simulink model "atrias_original"  (R2017a)
settings: Solver=ode45  StartTime=0.0  StopTime=sim_t  RelTol=1e-6  EnableMultiTasking=on
values from neighbouring files (symbols this model uses):
  N = grid_slice*1000    [createGrid.m]
  nm = fn_set_vnmc_params(sm, sample_time)    [kernel_scores_NM_mismatch.m]    (also in main_ATRIAS_cluster.m)
  nmc_BLCtrlPar = nmc.BLCtrlPar    [kernel_scores_NM_mismatch.m]    (also in main_ATRIAS_cluster.m)
  nmc_FPCtrlPar = nmc.FPCtrlPar    [kernel_scores_NM_mismatch.m]    (also in main_ATRIAS_cluster.m)
  nmc_LLCtrlPar = nmc.LLCtrlPar    [kernel_scores_NM_mismatch.m]    (also in main_ATRIAS_cluster.m)
  nmc_StCtrlPar = nmc.StCtrlPar    [kernel_scores_NM_mismatch.m]    (also in main_ATRIAS_cluster.m)
  nmc_SwCtrlPar = nmc.SwCtrlPar    [kernel_scores_NM_mismatch.m]    (also in main_ATRIAS_cluster.m)
  nmc_TrCtrlPar = nmc.TrCtrlPar    [kernel_scores_NM_mismatch.m]    (also in main_ATRIAS_cluster.m)
  nStep_switchCtrl = 10    [main_ATRIAS_cluster.m]
  nStep_thr = 1000    [createSimInitial.m]    (also in main_ATRIAS_cluster.m)
  rc_CtrlPar = [rc.k_placement, rc.T_step, rc.Cd, rc.kpt, rc.kdt, rc.desired_theta, rc.desired_z, rc.kpz, rc.kdz]    [kernel_scores_NM_mismatch.m]    (also in main_ATRIAS_cluster.m)
  sm = fn_set_MechParams(sm)    [kernel_scores_NM_mismatch.m]    (also in main_ATRIAS_cluster.m = fn_set_MechParams(sm,perturb))
  test_VNMC = 1    [createSimInitial.m]    (also in main_ATRIAS_cluster.m = 0)
undefined symbols (not defined in the file or in its folder): delta_phi_max, delta_phi_max_buffer, delta_phi_min, DiscIntNeverNeededParam, Discrete, idc, initial_dx_estimate, initial_dy_estimate, initial_dz_estimate, initial_z_estimate, kd_shin_max, kd_shin_min, kd_splay_max, kd_splay_min, kd_thigh_max, kd_thigh_min, kp_shin_max, kp_shin_min, kp_splay_max, kp_splay_min, kp_thigh_max, kp_thigh_min, mc, min_splay_angle, min_splay_buffer, phi_shin_max, phi_shin_max_buffer, phi_shin_min, phi_shin_min_buffer, phi_thigh_max, phi_thigh_max_buffer, phi_thigh_min, phi_thigh_min_buffer, rad, rc, s, sample_time, sgn, sim_d, t_friction, Time, X, Y, Z
libraries: sm_lib x202, nesl_utility x122, simulink x77, simulink_extras x24, fl_lib x16, mblibv1 x4, ctrlSharedLib x4, commnoisgen2 x1, dspswit3 x1
(part 6 of 17)

== system atrias_original/control/RC control/State Estimation ==
  Right or Left [1/0] : Inport
  Torso Roll [rad rad/s] : Inport  Port=2
  Torso Pitch [rad rad/s] : Inport  Port=3
  Torso Yaw [rad rad/s] : Inport  Port=4
  Left Leg Sagittal Angle [rad rad/s] : Inport  Port=5
  Left Leg Roll [rad rad/s] : Inport  Port=6
  Left Leg Length [m m/s] : Inport  Port=7
  Right Leg Sagittal Angle [rad rad/s] : Inport  Port=8
  Right Leg Roll [rad rad/s] : Inport  Port=9
  Right Leg Length [m m/s] : Inport  Port=10
  Enable Kalman Filtering [1/0] : Inport  Port=11
  Right GRF [X Z] [N N] : Inport  Port=12
  Left GRF [X Z] [N N] : Inport  Port=13
  " Acceleration Measurement [m/s^2] x3" : Inport  Port=14
  Entering Stance [1/0] : Inport  Port=15
  Demux : Demux  Outputs=2
  Demux{1..7} (7 alike) : Demux  Outputs=3
  Demux11 : Demux  Outputs=2
  Demux8 : Demux  Outputs=2
  Discrete-Time Integrator : DiscreteIntegrator  InitialConditionSetting=State (most efficient)  SampleTime=-1  ICPrevOutput=DiscIntNeverNeededParam  ICPrevScaledInput=DiscIntNeverNeededParam
  From3 : From  Commented=on  GotoTag=RightLeftPrimary
  Gain : Gain  Gain=[1 1 0 1 1 0 1 1 0]
  Kalman Filtering : Subsystem
  Logical Operator1 : Logic  Operator=NOT  AllPortsSameDT=off  OutDataTypeStr=boolean
  Mux{,1,3,5,8..9,11..12} (8 alike) : Mux  Inputs=3
  Mux{2,4,6,10,13..20} (12 alike) : Mux  Inputs=2
  PositionUsingRobotGeometry : MATLAB Function  TreatAsAtomicUnit=on
  Product3 : Product
  Product4 : Product
  Selector : Selector  InputPortWidth=2  IndexOptions=Index vector (dialog)  Indices=[2]  OutputSizes=1
  Selector1 : Selector  InputPortWidth=2  IndexOptions=Index vector (dialog)  Indices=[2]  OutputSizes=1
  Selector2 : Selector  InputPortWidth=2  IndexOptions=Index vector (dialog)  Indices=[2]  OutputSizes=1
  Sum : Sum  Inputs=|++
  Switch : Switch  Criteria=u2 ~= 0
  Switch1 : Switch  Criteria=u2 ~= 0
  Switch2 : Switch  Criteria=u2 ~= 0
  Switch3 : Switch  Commented=on  Criteria=u2 ~= 0
  Terminator6 : Terminator
  X Kalman Output : Scope  NumInputPorts=3
  Y Kalman Output : Scope  NumInputPorts=3
  Z Kalman Output : Scope  NumInputPorts=3
  "[ddx, ddy, ddz]" : Selector  InputPortWidth=9  IndexOptions=Index vector (dialog)  Indices=[3 6 9]  OutputSizes=1
  "[x dx]" : Selector  InputPortWidth=9  IndexOptions=Index vector (dialog)  Indices=[1 2]  OutputSizes=1
  "[y dy]" : Selector  InputPortWidth=9  IndexOptions=Index vector (dialog)  Indices=[4 5]  OutputSizes=1
  "[z dz]" : Selector  InputPortWidth=9  IndexOptions=Index vector (dialog)  Indices=[7 8]  OutputSizes=1
  body frame : Selector  InputPortWidth=9  IndexOptions=Index vector (dialog)  Indices=[1 2 3]  OutputSizes=1
  body frame1 : Selector  InputPortWidth=9  IndexOptions=Index vector (dialog)  Indices=[1 2 3]  OutputSizes=1
  body frame{2..9} (8 alike) : Selector  InputPortWidth=9  IndexOptions=Index vector (dialog)  Indices=[4 5 6]  OutputSizes=1
  "Horizontal COM [m, m/s]" : Outport
  "Lateral COM [m, m/s]" : Outport  Port=2
  "Vertical COM [m, m/s]" : Outport  Port=3
  Pelvis to COM Position [m m m] : Outport  Port=4
  Pelvis to COM Velocity [m/s m/s m/s] : Outport  Port=5
  Primary Foot to COM Position [m m m] : Outport  Port=6
  Primary Foot to COM Velocity [m/s m/s m/s] : Outport  Port=7
  COM Acceleration [m/s^2] x3 : Outport  Port=8
  Secondary to COM Position [m m m] : Outport  Port=9  PortDimensions=3
  Secondary to COM Velocity [m/s m/s m/s] : Outport  Port=10  PortDimensions=3
  wires:
  Discrete-Time Integrator/1 -> Mux11/3
  Demux5/3 -> Mux12/1, Discrete-Time Integrator/1
  Demux5/2 -> Mux11/1
  Demux5/1 -> Mux13/1
  Demux4/3 -> Mux12/2
  Mux11/1 -> X Kalman Output/2
  Demux4/1 -> Mux13/2
  Demux4/2 -> Mux11/2
  Mux13/1 -> X Kalman Output/1
  Mux12/1 -> X Kalman Output/3
  Mux9/1 -> Mux3/2, Demux7/1, Kalman Filtering/10("Initial [y, dy, ddy] [m, m/s, m/s^2]")
  Mux8/1 -> Mux3/1, Demux5/1, Kalman Filtering/9("Initial [x, dx, ddx] [m, m/s, m/s^2]")
  "[ddx, ddy, ddz]"/1 -> COM Acceleration [m/s^2] x3/1
  Mux3/1 -> Gain/1
  Demux2/2 -> Mux9/3
  Demux2/1 -> Mux8/3
  Demux2/3 -> Mux/3
  " Acceleration Measurement [m/s^2] x3"/1 -> Demux2/1, Kalman Filtering/12(COM XYZ Acceleration [m/s^2] x3)
  Left Leg Sagittal Angle [rad rad/s]/1 -> PositionUsingRobotGeometry/5(left_leg_sagittal_angle)
  Left Leg Roll [rad rad/s]/1 -> PositionUsingRobotGeometry/6(left_leg_lateral_angle)
  Left Leg Length [m m/s]/1 -> PositionUsingRobotGeometry/7(left_leg_length)
  Right Leg Sagittal Angle [rad rad/s]/1 -> PositionUsingRobotGeometry/8(right_leg_sagittal_angle)
  Right Leg Roll [rad rad/s]/1 -> PositionUsingRobotGeometry/9(right_leg_lateral_angle)
  Right Leg Length [m m/s]/1 -> PositionUsingRobotGeometry/10(right_leg_length)
  Right or Left [1/0]/1 -> [RightLeftPrimary], PositionUsingRobotGeometry/1(right_left)
  Torso Roll [rad rad/s]/1 -> PositionUsingRobotGeometry/2(roll)
  Torso Yaw [rad rad/s]/1 -> PositionUsingRobotGeometry/4(yaw)
  Torso Pitch [rad rad/s]/1 -> PositionUsingRobotGeometry/3(pitch)
  Mux5/1 -> Switch/1
  Selector/1 -> Kalman Filtering/7(Right Vertical GRF [N])
  Selector1/1 -> Kalman Filtering/8(Left Vertical GRF [N])
  Product4/1 -> Sum/2, Selector1/1
  Product3/1 -> Sum/1, Selector/1
  Sum/1 -> Demux/1
  Enable Kalman Filtering [1/0]/1 -> Kalman Filtering/Enable, [EnableKalmanFiltering]
  Demux/1 -> Kalman Filtering/5(GRFx [N])
  Mux1/1 -> Terminator6/1
  PositionUsingRobotGeometry/12(dcom_pelvis) -> body frame1/1
  PositionUsingRobotGeometry/11(com_pelvis) -> body frame/1
  body frame/1 -> Pelvis to COM Position [m m m]/1
  body frame1/1 -> Pelvis to COM Velocity [m/s m/s m/s]/1
  PositionUsingRobotGeometry/7(lateral_com_position) -> Mux9/1
  "[z dz]"/1 -> "Vertical COM [m, m/s]"/1
  Switch/1 -> "[x dx]"/1, "[y dy]"/1, "[z dz]"/1, "[ddx, ddy, ddz]"/1
  "[y dy]"/1 -> "Lateral COM [m, m/s]"/1
  Demux/2 -> Kalman Filtering/6(GRFz [N])
  Kalman Filtering/1("[x, dx, ddx] [m/s, m/s^2]") -> Mux5/1, Demux4/1
  Kalman Filtering/3("[z, dz, ddz] [m, m/s, m/s^2]") -> Demux1/1, Mux5/3
  Kalman Filtering/2("[y, dy, ddy] [m/s, m/s^2]") -> Demux6/1, Mux5/2
  Kalman Filtering/5("[y, dy, ddy] uncertainty") -> Mux1/2
  Kalman Filtering/4("[x, dx, ddx] uncertainty") -> Mux1/1
  Kalman Filtering/6("[z, dz, ddz] uncertainty") -> Mux1/3
  PositionUsingRobotGeometry/9(vertical_com_position) -> Mux/1
  PositionUsingRobotGeometry/10(vertical_com_velocity) -> Mux/2
  Mux/1 -> Mux3/3, Demux3/1, Kalman Filtering/11("Initial [z, dz, ddz] [m m/s m/s^2]")
  PositionUsingRobotGeometry/8(lateral_com_velocity) -> Mux9/2
  PositionUsingRobotGeometry/6(horizontal_com_velocity) -> Mux8/2
  [RightLeftPrimary] -> Switch2/2
  Mux17/1 -> Switch2/3
  Mux16/1 -> Switch2/1
  Switch2/1 -> Demux11/1
  Demux11/2 -> Primary Foot to COM Velocity [m/s m/s m/s]/1
  Demux11/1 -> Primary Foot to COM Position [m m m]/1
  body frame2/1 -> Mux17/1
  body frame3/1 -> Mux17/2
  body frame5/1 -> Mux16/2
  body frame4/1 -> Mux16/1
  Entering Stance [1/0]/1 -> Kalman Filtering/13(Entering Stance [1/0])
  Mux4/1 -> Z Kalman Output/3
  Mux6/1 -> Z Kalman Output/1
  Demux1/2 -> Mux10/2
  Demux1/1 -> Mux6/2
  Mux10/1 -> Z Kalman Output/2
  Demux1/3 -> Mux4/2
  Demux3/1 -> Mux6/1
  Demux3/2 -> Mux10/1
  Demux3/3 -> Mux4/1
  Mux15/1 -> Y Kalman Output/3
  Mux18/1 -> Y Kalman Output/1
  Demux6/2 -> Mux14/2
  Demux6/1 -> Mux18/2
  Mux14/1 -> Y Kalman Output/2
  Demux6/3 -> Mux15/2
  Demux7/1 -> Mux18/1
  Demux7/2 -> Mux14/1
  Demux7/3 -> Mux15/1
  [EnableKalmanFiltering] -> Switch/2
  PositionUsingRobotGeometry/1(com_left_foot) -> body frame8/1, body frame2/1, Kalman Filtering/1("COM from Left Foot [body, yawed, global]")
  PositionUsingRobotGeometry/2(dcom_left_foot) -> body frame9/1, body frame3/1, Kalman Filtering/2("dCOM from Left Foot [body, yawed, global]")
  PositionUsingRobotGeometry/3(com_right_foot) -> body frame6/1, body frame4/1, Kalman Filtering/3("COM from Right Foot [body, yawed, global]")
  PositionUsingRobotGeometry/4(dcom_right_foot) -> Kalman Filtering/4("dCOM from Right Foot [body, yawed, global]"), body frame7/1, body frame5/1
  [RightLeftPrimary] -> Switch1/2
  Mux20/1 -> Switch1/3
  Mux19/1 -> Switch1/1
  Switch1/1 -> Demux8/1
  Demux8/2 -> Secondary to COM Velocity [m/s m/s m/s]/1
  Demux8/1 -> Secondary to COM Position [m m m]/1
  body frame6/1 -> Mux20/1
  body frame7/1 -> Mux20/2
  body frame9/1 -> Mux19/2
  body frame8/1 -> Mux19/1
  Gain/1 -> Switch/3
  From3/1 -> Switch3/2
  Logical Operator1/1 -> Product4/1
  Left GRF [X Z] [N N]/1 -> Product4/2
  Right GRF [X Z] [N N]/1 -> Product3/2
  [RightLeftPrimary] -> Logical Operator1/1, Product3/1
  Mux2/1 -> "Horizontal COM [m, m/s]"/1
  Selector2/1 -> Mux2/2
  "[x dx]"/1 -> Selector2/1
  PositionUsingRobotGeometry/5(horizontal_com_position) -> Mux2/1, Mux8/1

== system atrias_original/control/RC control/Step Count ==
  In1 : Inport
  Data Type Conversion : DataTypeConversion  OutDataTypeStr=uint32
  Sum1 : Sum  Inputs=|++
  Unit Delay : UnitDelay  SampleTime=-1
  step count : Scope
  Out1 : Outport
  wires:
  In1/1 -> Data Type Conversion/1
  Unit Delay/1 -> Sum1/2
  Sum1/1 -> Out1/1, Unit Delay/1, step count/1
  Data Type Conversion/1 -> Sum1/1

== system atrias_original/control/RC control/Swing ==
  desired_x : Inport
  EnteringStance : Inport  Port=2
  nstep : Inport  Port=3
  secondary_x : Inport  Port=4
  tSim : Inport  Port=5
  T_step : Inport  Port=6
  Enabled Subsystem : Subsystem  TreatAsAtomicUnit=on
  Hold Value1 : Subsystem  TreatAsAtomicUnit=on
  Sum5 : Sum  Inputs=|-+
  To Workspace1 : ToWorkspace  VariableName=nStep  SampleTime=-1
      settings: MaxDataPoints=1  Save2DSignal=2-D array (concatenate along first dimension)
  Unit Delay1 : UnitDelay  InitialCondition=0.4  SampleTime=sample_time
  swing_trajectory_regenerator : MATLAB Function  TreatAsAtomicUnit=on
  x : Outport
  xd : Outport  Port=2
  xdd : Outport  Port=3
  z : Outport  Port=4
  zd : Outport  Port=5
  zdd : Outport  Port=6
  tStance_last : Outport  Port=7
  wires:
  swing_trajectory_regenerator/2(xd) -> xd/1
  Unit Delay1/1 -> Hold Value1/1(In1)
  nstep/1 -> To Workspace1/1, swing_trajectory_regenerator/4(nstep)
  swing_trajectory_regenerator/1(x) -> x/1
  EnteringStance/1 -> Hold Value1/Enable, Enabled Subsystem/Enable
  Hold Value1/1(Out1) -> tStance_last/1
  swing_trajectory_regenerator/4(z) -> z/1
  desired_x/1 -> swing_trajectory_regenerator/5(x1)
  swing_trajectory_regenerator/5(zd) -> zd/1
  Enabled Subsystem/1(Out1) -> Sum5/1
  secondary_x/1 -> swing_trajectory_regenerator/3(x0)
  tSim/1 -> Enabled Subsystem/1(In1), Sum5/2
  swing_trajectory_regenerator/6(zdd) -> zdd/1
  swing_trajectory_regenerator/3(xdd) -> xdd/1
  Sum5/1 -> [time_step]
  [time_step] -> Unit Delay1/1
  [time_step] -> swing_trajectory_regenerator/2(time_step)
  T_step/1 -> swing_trajectory_regenerator/1(T_step)

== system atrias_original/control/RC control/Torque Distribution ==
  Leg Force [N] : Inport
  Leg Torque [Nm] : Inport  Port=2
  Primary Leg Width [m] : Inport  Port=3
  Gain : Gain  Gain=0.5
  Gain1 : Gain  Gain=0.5
  Motor Torque Saturation Optimization : MATLAB Function  Commented=on  TreatAsAtomicUnit=on
  Product : Product  RndMeth=Zero
  Sum : Sum  Inputs=|++
  Sum1 : Sum  Inputs=+-|
  Back Torque [Nm] : Outport
  Front Torque [Nm] : Outport  Port=2
  wires:
  Sum1/1 -> Back Torque [Nm]/1
  Leg Torque [Nm]/1 -> Gain/1
  Sum/1 -> Front Torque [Nm]/1
  Gain/1 -> Sum/1, Sum1/1
  Primary Leg Width [m]/1 -> Product/2
  Gain1/1 -> Sum1/2, Sum/2
  Leg Force [N]/1 -> Product/1
  Product/1 -> Gain1/1

== system atrias_original/control/RC control/lateralControl2D ==
  Primary Axial Leg Force [N] : Inport
  desired_SecondaryLegRoll : Inport  Port=2
  SecondaryLegRoll : Inport  Port=3
  RightLeftPrimary [1 or 0] : Inport  Port=4
  2D Lateral Stance Control : MATLAB Function  TreatAsAtomicUnit=on
  Mux : Mux  Inputs=2
  Mux1 : Mux  Inputs=2
  Primary Lateral Torque Saturation : Saturate  UpperLimit=mc.max_primary_lateral_stance_torque  LowerLimit=-mc.max_primary_lateral_stance_torque
      settings: AttributesFormatString=Top: %<UpperLimit>\nBottom: %<LowerLimit>
  Switch : Switch  Criteria=u2 ~= 0
  Lateral Torque command [R L] : Outport
  wires:
  2D Lateral Stance Control/1(tau_primary) -> Primary Lateral Torque Saturation/1
  Primary Lateral Torque Saturation/1 -> Mux1/2, Mux/1
  Primary Axial Leg Force [N]/1 -> 2D Lateral Stance Control/1(F_leg)
  2D Lateral Stance Control/2(tau_secondary) -> Mux1/1, Mux/2
  desired_SecondaryLegRoll/1 -> 2D Lateral Stance Control/2(desired_SecondaryLegRoll)
  SecondaryLegRoll/1 -> 2D Lateral Stance Control/3(SecondaryLegRoll)
  RightLeftPrimary [1 or 0]/1 -> Switch/2
  Switch/1 -> Lateral Torque command [R L]/1
  Mux/1 -> Switch/1
  Mux1/1 -> Switch/3

== system atrias_original/control/RC control/lateral_PID_control ==
  Desired Lateral State [rad rad/s] : Inport
  Secondary Leg Roll Position [rad] : Inport  Port=2
  Secondary Leg Roll Velocity [rad/s] : Inport  Port=3
  q_boom_roll : Inport  Port=4
  Right Left Primary [1 or 0] : Inport  Port=5
  q_lateral [R L] : Inport  Port=6
  dq_lateral [R L] : Inport  Port=7
  Demux : Demux  Outputs=2
  Demux1 : Demux  Outputs=2
  Gain : Gain  Gain=-1
  Gain2 : Gain  Gain=-1
  Lateral Hip PID1 : Subsystem
  Mux : Mux  Inputs=2
  Mux1 : Mux  Inputs=2
  Mux3 : Mux  Inputs=2
  Sum{1..3,5} (4 alike) : Sum  Inputs=|+-
  Sum4 : Sum  Inputs=++|
  Sum6 : Sum  Inputs=++|
  Swing Leg Lateral : Subsystem
  Switch : Switch  Criteria=u2 ~= 0
  Switch1 : Switch  Criteria=u2 ~= 0
  Torque Saturation : Saturate  UpperLimit=mc.max_torque_lateral  LowerLimit=-mc.max_torque_lateral  ZeroCross=off
      settings: AttributesFormatString=Top: %<UpperLimit>\nBottom: %<LowerLimit>
  desired_velocity : Constant  Value=0
  feedforward_torque (gravity compensation) : Constant  Value=mc.hip_gravity_compensation
  feedforward_torque (gravity compensation)1 : Constant  Value=mc.hip_gravity_compensation
  spherical_correction_angle : Subsystem
  tau_lateral [R L] : Outport
  wires:
  Desired Lateral State [rad rad/s]/1 -> Demux/1
  Secondary Leg Roll Position [rad]/1 -> Sum2/2
  feedforward_torque (gravity compensation)/1 -> Sum4/1
  Sum1/1 -> Swing Leg Lateral/2(velocity_error)
  Demux/2 -> Sum1/1
  Secondary Leg Roll Velocity [rad/s]/1 -> Sum1/2
  Sum2/1 -> Swing Leg Lateral/1(position_error)
  Swing Leg Lateral/1(out) -> Sum4/2
  Demux/1 -> Sum2/1
  spherical_correction_angle/1(lateral_correction [rad]) -> Mux/1, Gain/1
  Gain/1 -> Mux/2
  q_boom_roll/1 -> spherical_correction_angle/1(q_boom_roll)
  q_lateral [R L]/1 -> Sum5/2
  Sum3/1 -> Lateral Hip PID1/2(velocity_error)
  dq_lateral [R L]/1 -> Sum3/2
  Sum5/1 -> Lateral Hip PID1/1(position_error)
  Sum6/1 -> Gain2/1
  feedforward_torque (gravity compensation)1/1 -> Sum6/1
  Lateral Hip PID1/1(out) -> Sum6/2
  Switch/1 -> Torque Saturation/1
  Mux/1 -> Sum5/1
  desired_velocity/1 -> Sum3/1
  Torque Saturation/1 -> tau_lateral [R L]/1
  Switch1/1 -> Mux3/2, Mux1/1
  Sum4/1 -> Mux3/1, Mux1/2
  Right Left Primary [1 or 0]/1 -> Switch1/2, Switch/2
  Mux1/1 -> Switch/1
  Mux3/1 -> Switch/3
  Demux1/1 -> Switch1/1
  Demux1/2 -> Switch1/3
  Gain2/1 -> Demux1/1

== system atrias_original/control/Robot-to-NMM Interface/Contact State Machine ==
  Contact Factor [body weight] : Inport
  "[Z dZ] [m m/s]" : Inport  Port=2
  ddZ [m/s^2] : Inport  Port=3
  Detect Increase : simulink/Logic and Bit Operations/Detect Increase  vinit=1.0  InputProcessing=Inherited  OutDataTypeStr=boolean
  Detect Fall Nonpositive : simulink/Logic and Bit Operations/Detect Fall Nonpositive  vinit=1  InputProcessing=Inherited  OutDataTypeStr=boolean
      settings: SourceProductName=Simulink  SourceProductBaseCode=SL
  Mux25 : Mux
  Selector : Selector  InputPortWidth=2  IndexOptions=Index vector (dialog)  Indices=[2]  OutputSizes=1
  State Machine : State Transition Table  TreatAsAtomicUnit=on
  Terminator8 : Terminator
  Unit Delay1 : UnitDelay  InitialCondition=1  SampleTime=sample_time
  Unit Delay5 : UnitDelay  SampleTime=-1
  Unit Delay6 : UnitDelay  SampleTime=sample_time
  Unit Delay7 : UnitDelay  InitialCondition=1  SampleTime=sample_time
  Unit Delay8 : UnitDelay  SampleTime=sample_time
  flight [1/0] : Outport
  Exiting Stance [1/0] : Outport  Port=2
  Entering stance [1/0] : Outport  Port=3
  wires:
  ddZ [m/s^2]/1 -> State Machine/4(vertical_acceleration)
  "[Z dZ] [m m/s]"/1 -> Selector/1
  Mux25/1 -> Unit Delay8/1
  State Machine/4(" Flight") -> Mux25/4, Unit Delay7/1
  Unit Delay5/1 -> State Machine/2(previous_z_velocity)
  Contact Factor [body weight]/1 -> State Machine/3(vertical_grf)
  Selector/1 -> Unit Delay5/1, State Machine/1(z_velocity)
  Unit Delay8/1 -> Terminator8/1
  Unit Delay6/1 -> Detect Fall Nonpositive/1
  Unit Delay7/1 -> flight [1/0]/1
  Detect Fall Nonpositive/1 -> Exiting Stance [1/0]/1
  State Machine/1(" TouchDown") -> Unit Delay1/1, Mux25/1
  Detect Increase/1 -> Entering stance [1/0]/1
  Unit Delay1/1 -> Detect Increase/1
  State Machine/3(" Takeoff") -> Unit Delay6/1, Mux25/3
  State Machine/2(" Unloading") -> Mux25/2

== system atrias_original/control/Robot-to-NMM Interface/Contact State Machine1 ==
  Contact Factor [body weight] : Inport
  "[Z dZ] [m m/s]" : Inport  Port=2
  ddZ [m/s^2] : Inport  Port=3
  Detect Increase : simulink/Logic and Bit Operations/Detect Increase  vinit=1.0  InputProcessing=Inherited  OutDataTypeStr=boolean
  Detect Fall Nonpositive : simulink/Logic and Bit Operations/Detect Fall Nonpositive  vinit=1  InputProcessing=Inherited  OutDataTypeStr=boolean
      settings: SourceProductName=Simulink  SourceProductBaseCode=SL
  Mux25 : Mux
  Selector : Selector  InputPortWidth=2  IndexOptions=Index vector (dialog)  Indices=[2]  OutputSizes=1
  State Machine : State Transition Table  TreatAsAtomicUnit=on
  Terminator8 : Terminator
  Unit Delay1 : UnitDelay  InitialCondition=1  SampleTime=sample_time
  Unit Delay5 : UnitDelay  SampleTime=-1
  Unit Delay6 : UnitDelay  SampleTime=sample_time
  Unit Delay7 : UnitDelay  InitialCondition=1  SampleTime=sample_time
  Unit Delay8 : UnitDelay  SampleTime=sample_time
  flight [1/0] : Outport
  Exiting Stance [1/0] : Outport  Port=2
  Entering stance [1/0] : Outport  Port=3
  wires:
  ddZ [m/s^2]/1 -> State Machine/4(vertical_acceleration)
  "[Z dZ] [m m/s]"/1 -> Selector/1
  Mux25/1 -> Unit Delay8/1
  State Machine/4(" Flight") -> Mux25/4, Unit Delay7/1
  Unit Delay5/1 -> State Machine/2(previous_z_velocity)
  Contact Factor [body weight]/1 -> State Machine/3(vertical_grf)
  Selector/1 -> Unit Delay5/1, State Machine/1(z_velocity)
  Unit Delay8/1 -> Terminator8/1
  Unit Delay6/1 -> Detect Fall Nonpositive/1
  Unit Delay7/1 -> flight [1/0]/1
  Detect Fall Nonpositive/1 -> Exiting Stance [1/0]/1
  State Machine/1(" TouchDown") -> Unit Delay1/1, Mux25/1
  Detect Increase/1 -> Entering stance [1/0]/1
  Unit Delay1/1 -> Detect Increase/1
  State Machine/3(" Takeoff") -> Unit Delay6/1, Mux25/3
  State Machine/2(" Unloading") -> Mux25/2

== system atrias_original/control/Robot-to-NMM Interface/Force Estimation ==
  q : Inport
  Torso Pitch [rad] : Inport  Port=2
  Right/Left Primary : Inport  Port=3
  Leg Angle Right/Left [rad rad] : Inport  Port=4
  Leg Width Right/Left [m m] : Inport  Port=5
  Leg Length Right/Left [m m] : Inport  Port=6
  Constant13 : Constant  Value=mc.m_total_real*mc.g
  Demux{,1,19..20} (4 alike) : Demux  Outputs=2
  Divide : Product  Inputs=*/
  Horizontal GRF : Subsystem
  Leg Force Measurements : Subsystem
  Leg Plane GRF : Subsystem
  Mux{,1..3} (4 alike) : Mux  Inputs=2
  Saturation : Saturate  UpperLimit=Inf  LowerLimit=0
  Sum11 : Sum  Inputs=|++
  Switch1 : Switch  Criteria=u2 ~= 0
  two_pole_filter : DiscreteTransferFcn  Numerator=[(1-2*exp(-mc.fcut_contact*sample_time)+exp(-2*mc.fcut_contact*sample_time)) 0 0]  Denominator=[1 (-2*exp(-mc.fcut_contact*sample_time)) (exp(-2*mc.fcut_contact*sample_time))]  SampleTime=sample_time
  Vertical GRF [body weight] : Outport
  Right Leg Measured Axial Force [N] : Outport  Port=2
  Left Leg Measured Axial Force [N] : Outport  Port=3
  Primary Measured Vertical GRF [N] : Outport  Port=4
  "Right [horizontal GRF, vertical GRF] [N N]" : Outport  Port=5
  "Left [horizontal GRF, vertical GRF] [N N]" : Outport  Port=6
  GRFx : Outport  Port=7
  wires:
  Divide/1 -> Vertical GRF [body weight]/1
  Leg Width Right/Left [m m]/1 -> Leg Force Measurements/2(Leg Width Right/Left [m m])
  q/1 -> Leg Force Measurements/1(q)
  two_pole_filter/1 -> Divide/1
  Constant13/1 -> Divide/2
  Right/Left Primary/1 -> Switch1/2
  Leg Length Right/Left [m m]/1 -> Leg Force Measurements/3(Leg Length Right/Left [m m])
  Leg Force Measurements/3(Right Leg Axial Force [N]) -> Right Leg Measured Axial Force [N]/1, Mux/1
  Leg Force Measurements/4(Left Leg Axial Force [N]) -> Left Leg Measured Axial Force [N]/1, Mux/2
  Mux1/1 -> Leg Plane GRF/2(Orthogonal Force [N]), Horizontal GRF/2(Orthogonal Force [N])
  Torso Pitch [rad]/1 -> Leg Plane GRF/3(Torso Pitch [rad]), Horizontal GRF/3(Torso Pitch [rad])
  Switch1/1 -> Primary Measured Vertical GRF [N]/1, two_pole_filter/1
  Demux/1 -> Mux2/2, Switch1/1
  Demux/2 -> Mux3/2, Switch1/3
  Leg Angle Right/Left [rad rad]/1 -> Leg Plane GRF/4(Leg Angle [rad]), Horizontal GRF/4(Leg Angle [rad])
  Horizontal GRF/1(Horizontal Force [N]) -> Demux1/1
  Mux/1 -> Leg Plane GRF/1(Axial Force [N]), Horizontal GRF/1(Axial Force [N])
  Demux1/1 -> Mux2/1
  Demux1/2 -> Mux3/1
  Saturation/1 -> Demux/1
  Mux2/1 -> Demux19/1, "Right [horizontal GRF, vertical GRF] [N N]"/1
  Mux3/1 -> Demux20/1, "Left [horizontal GRF, vertical GRF] [N N]"/1
  Demux19/1 -> Sum11/1
  Demux20/1 -> Sum11/2
  Sum11/1 -> GRFx/1
  Leg Force Measurements/5(Right Leg Orthogonal Force [N]) -> Mux1/1
  Leg Force Measurements/6(Left Leg Orthogonal Force [N]) -> Mux1/2
  Leg Plane GRF/1(Vertical Force [N]) -> Saturation/1

== system atrias_original/control/Robot-to-NMM Interface/L Leg Calculator ==
  Front [rad rad/s] : Inport
  Back [rad rad/s] : Inport  Port=2
  Demux1 : Demux  Outputs=2
  Gain1 : Gain  Gain=2*mc.l_seg
  Gain2 : Gain  Gain=mc.l_seg
  Gain3 : Gain  Gain=-1
  Gain4 : Gain  Gain=0.5
  Gain5 : Gain  Gain=0.5
  Gain6 : Gain  Gain=2
  Mux1 : Mux  Inputs=2
  Product : Product  RndMeth=Zero
  Sum4 : Sum  Inputs=+|+
  Sum5 : Sum  Inputs=+|-
  Trigonometric Function : Trigonometry  Operator=cos
  Trigonometric Function1 : Trigonometry
  "Leg Length [m m/s] " : Outport
  Leg Angle [rad rad/s] : Outport  Port=2
  Leg Splay [rad rad/s] : Outport  Port=3
  Leg Width [m] : Outport  Port=4
  wires:
  Gain6/1 -> Leg Width [m]/1
  Gain4/1 -> Trigonometric Function1/1, Trigonometric Function/1
  Trigonometric Function/1 -> Gain1/1
  Gain1/1 -> Mux1/1
  Trigonometric Function1/1 -> Gain2/1
  Product/1 -> Mux1/2
  Front [rad rad/s]/1 -> Sum5/2, Sum4/2
  Back [rad rad/s]/1 -> Sum4/1, Sum5/1
  Demux1/2 -> Gain3/1
  Gain3/1 -> Product/2
  Demux1/1 -> Gain4/1
  Gain2/1 -> Product/1, Gain6/1
  Sum5/1 -> Leg Splay [rad rad/s]/1, Demux1/1
  Mux1/1 -> "Leg Length [m m/s] "/1
  Sum4/1 -> Gain5/1
  Gain5/1 -> Leg Angle [rad rad/s]/1

== system atrias_original/control/Robot-to-NMM Interface/R Leg Calculator ==
  Front [rad rad/s] : Inport
  Back [rad rad/s] : Inport  Port=2
  Demux1 : Demux  Outputs=2
  Gain1 : Gain  Gain=2*mc.l_seg
  Gain2 : Gain  Gain=mc.l_seg
  Gain3 : Gain  Gain=-1
  Gain4 : Gain  Gain=0.5
  Gain5 : Gain  Gain=0.5
  Gain6 : Gain  Gain=2
  Mux1 : Mux  Inputs=2
  Product : Product  RndMeth=Zero
  Sum4 : Sum  Inputs=+|+
  Sum5 : Sum  Inputs=+|-
  Trigonometric Function : Trigonometry  Operator=cos
  Trigonometric Function1 : Trigonometry
  "Leg Length [m m/s] " : Outport
  Leg Angle [rad rad/s] : Outport  Port=2
  Leg Splay [rad rad/s] : Outport  Port=3
  Leg Width [m] : Outport  Port=4
  wires:
  Gain5/1 -> Leg Angle [rad rad/s]/1
  Sum4/1 -> Gain5/1
  Mux1/1 -> "Leg Length [m m/s] "/1
  Sum5/1 -> Demux1/1, Leg Splay [rad rad/s]/1
  Gain2/1 -> Gain6/1, Product/1
  Demux1/1 -> Gain4/1
  Gain3/1 -> Product/2
  Demux1/2 -> Gain3/1
  Back [rad rad/s]/1 -> Sum5/1, Sum4/1
  Front [rad rad/s]/1 -> Sum4/2, Sum5/2
  Product/1 -> Mux1/2
  Trigonometric Function1/1 -> Gain2/1
  Gain1/1 -> Mux1/1
  Trigonometric Function/1 -> Gain1/1
  Gain4/1 -> Trigonometric Function/1, Trigonometric Function1/1
  Gain6/1 -> Leg Width [m]/1

== system atrias_original/control/Robot-to-NMM Interface/R Leg Geometry f(l_seg, l_v, v12_max) ==
  qBack [rad] : Inport
  qFront [rad] : Inport  Port=2
  dqBack [rad/s] : Inport  Port=3
  dqFront [rad/s] : Inport  Port=4
  Constant : Constant  Value=pi/2
  Constant1 : Constant  Value=mc.l_seg/nm.l_v
  Divide : Product  Inputs=**/
  Fcn : Fcn  Expr=(1-u(3))/2*u(1) + (1+u(3))/2*u(2)
  Fcn1 : Fcn  Expr=-u(3)*u(1) + u(3)*u(2)
  Gain : Gain  Gain=0.5
  Gain1 : Gain  Gain=0.5
  Gain2 : Gain  Gain=mc.l_seg/nm.l_v
  Gain3 : Gain  Gain=2
  Gain4 : Gain  Gain=0.5
  Mux : Mux  Inputs=3
  Sum : Sum  Inputs=|+-
  Sum1 : Sum  Inputs=|+-
  Sum2 : Sum  Inputs=|++
  Sum3 : Sum  Inputs=|++
  Trigonometric Function : Trigonometry  Operator=cos
  Trigonometric Function1 : Trigonometry  Operator=asin
  Trigonometric Function2 : Trigonometry
  Trigonometric Function3 : Trigonometry  Operator=cos
  "[0,sin(v12_max/2)]" : Saturate  UpperLimit=sin(nm.v12_max/2)  LowerLimit=0
  "[0,v12_max]" : Saturate  UpperLimit=nm.v12_max  LowerLimit=0
  "[min_splay_angle/2, inf]" : Saturate  UpperLimit=inf  LowerLimit=nm.min_splay_angle/2
  virtual knee angle [rad] : Outport
  virtual knee velocity [rad/s] : Outport  Port=2
  virtual hip angle [rad] : Outport  Port=3
  virtual hip velocity [rad/s] : Outport  Port=4
  k : Outport  Port=5
  wires:
  Sum/1 -> Gain/1
  qBack [rad]/1 -> [qB]
  qFront [rad]/1 -> [qF]
  dqBack [rad/s]/1 -> [dqB]
  dqFront [rad/s]/1 -> [dqF]
  [qF] -> Sum3/2, Sum/2
  [qB] -> Sum/1, Sum3/1
  Gain/1 -> Trigonometric Function/1, "[min_splay_angle/2, inf]"/1
  [phiK] -> Gain1/1
  Sum1/1 -> Sum2/1
  Constant/1 -> Sum1/2
  Gain1/1 -> Trigonometric Function3/1, Sum2/2
  Sum2/1 -> [phiH]
  Trigonometric Function/1 -> Gain2/1
  Gain2/1 -> "[0,sin(v12_max/2)]"/1
  "[0,sin(v12_max/2)]"/1 -> Trigonometric Function1/1
  Trigonometric Function1/1 -> "[0,v12_max]"/1
  "[0,v12_max]"/1 -> Gain3/1
  Gain3/1 -> [phiK]
  [phiK] -> virtual knee angle [rad]/1
  [phiH] -> virtual hip angle [rad]/1
  Trigonometric Function2/1 -> Divide/2
  Constant1/1 -> Divide/1
  Trigonometric Function3/1 -> Divide/3
  Divide/1 -> k/1, Mux/3
  Mux/1 -> Fcn/1, Fcn1/1
  [dqF] -> Mux/2
  [dqB] -> Mux/1
  Fcn/1 -> virtual hip velocity [rad/s]/1
  Fcn1/1 -> virtual knee velocity [rad/s]/1
  Sum3/1 -> Gain4/1
  Gain4/1 -> Sum1/1
  "[min_splay_angle/2, inf]"/1 -> Trigonometric Function2/1

== system atrias_original/control/Robot-to-NMM Interface/R Leg Geometry f(l_seg, l_v, v12_max)1 ==
  qBack [rad] : Inport
  qFront [rad] : Inport  Port=2
  dqBack [rad/s] : Inport  Port=3
  dqFront [rad/s] : Inport  Port=4
  Constant : Constant  Value=pi/2
  Constant1 : Constant  Value=mc.l_seg/nm.l_v
  Divide : Product  Inputs=**/
  Fcn : Fcn  Expr=(1-u(3))/2*u(1) + (1+u(3))/2*u(2)
  Fcn1 : Fcn  Expr=-u(3)*u(1) + u(3)*u(2)
  Gain : Gain  Gain=0.5
  Gain1 : Gain  Gain=0.5
  Gain2 : Gain  Gain=mc.l_seg/nm.l_v
  Gain3 : Gain  Gain=2
  Gain4 : Gain  Gain=0.5
  Mux : Mux  Inputs=3
  Sum : Sum  Inputs=|+-
  Sum1 : Sum  Inputs=|+-
  Sum2 : Sum  Inputs=|++
  Sum3 : Sum  Inputs=|++
  Trigonometric Function : Trigonometry  Operator=cos
  Trigonometric Function1 : Trigonometry  Operator=asin
  Trigonometric Function2 : Trigonometry
  Trigonometric Function3 : Trigonometry  Operator=cos
  "[0,sin(v12_max/2)]" : Saturate  UpperLimit=sin(nm.v12_max/2)  LowerLimit=0
  "[0,v12_max]" : Saturate  UpperLimit=nm.v12_max  LowerLimit=0
  "[min_splay_angle/2, inf]" : Saturate  UpperLimit=inf  LowerLimit=nm.min_splay_angle/2
  virtual knee angle [rad] : Outport
  virtual knee velocity [rad/s] : Outport  Port=2
  virtual hip angle [rad] : Outport  Port=3
  virtual hip velocity [rad/s] : Outport  Port=4
  k : Outport  Port=5
  wires:
  "[min_splay_angle/2, inf]"/1 -> Trigonometric Function2/1
  Gain4/1 -> Sum1/1
  Sum3/1 -> Gain4/1
  Fcn1/1 -> virtual knee velocity [rad/s]/1
  Fcn/1 -> virtual hip velocity [rad/s]/1
  [dqB] -> Mux/1
  [dqF] -> Mux/2
  Mux/1 -> Fcn1/1, Fcn/1
  Divide/1 -> Mux/3, k/1
  Trigonometric Function3/1 -> Divide/3
  Constant1/1 -> Divide/1
  Trigonometric Function2/1 -> Divide/2
  [phiH] -> virtual hip angle [rad]/1
  [phiK] -> virtual knee angle [rad]/1
  Gain3/1 -> [phiK]
  "[0,v12_max]"/1 -> Gain3/1
  Trigonometric Function1/1 -> "[0,v12_max]"/1
  "[0,sin(v12_max/2)]"/1 -> Trigonometric Function1/1
  Gain2/1 -> "[0,sin(v12_max/2)]"/1
  Trigonometric Function/1 -> Gain2/1
  Sum2/1 -> [phiH]
  Gain1/1 -> Sum2/2, Trigonometric Function3/1
  Constant/1 -> Sum1/2
  Sum1/1 -> Sum2/1
  [phiK] -> Gain1/1
  Gain/1 -> "[min_splay_angle/2, inf]"/1, Trigonometric Function/1
  [qB] -> Sum3/1, Sum/1
  [qF] -> Sum/2, Sum3/2
  dqFront [rad/s]/1 -> [dqF]
  dqBack [rad/s]/1 -> [dqB]
  qFront [rad]/1 -> [qF]
  qBack [rad]/1 -> [qB]
  Sum/1 -> Gain/1

== system atrias_original/control/Robot-to-NMM Interface/RC Demux ==
  In1 : Inport
  Selector1 : Selector  InputPortWidth=13  IndexOptions=Index vector (dialog)  Indices=[10]  OutputSizes=1
  Selector18 : Selector  InputPortWidth=13  IndexOptions=Index vector (dialog)  Indices=[13]  OutputSizes=1
  Selector2 : Selector  InputPortWidth=13  IndexOptions=Index vector (dialog)  Indices=[5 6]  OutputSizes=1
  Selector23 : Selector  InputPortWidth=13  IndexOptions=Index vector (dialog)  Indices=[11]  OutputSizes=1
  Selector28 : Selector  InputPortWidth=13  IndexOptions=Index vector (dialog)  Indices=[12]  OutputSizes=1
  Selector4 : Selector  InputPortWidth=13  IndexOptions=Index vector (dialog)  Indices=[7 8]  OutputSizes=1
  Selector5 : Selector  InputPortWidth=13  IndexOptions=Index vector (dialog)  Indices=[9]  OutputSizes=1
  Selector6 : Selector  InputPortWidth=13  IndexOptions=Index vector (dialog)  Indices=[1 2]  OutputSizes=1
  Selector7 : Selector  InputPortWidth=13  IndexOptions=Index vector (dialog)  Indices=[3 4]  OutputSizes=1
  Out1 : Outport
  Out2 : Outport  Port=2
  Out3 : Outport  Port=3
  Out4 : Outport  Port=4
  Out5 : Outport  Port=5
  Out6 : Outport  Port=6
  Out7 : Outport  Port=7
  Out8 : Outport  Port=8
  Out9 : Outport  Port=9
  wires:
  Selector28/1 -> Out8/1
  Selector7/1 -> Out2/1
  Selector5/1 -> Out5/1
  Selector4/1 -> Out4/1
  Selector1/1 -> Out6/1
  In1/1 -> Selector1/1, Selector23/1, Selector28/1, Selector18/1, Selector5/1, Selector4/1, Selector2/1, Selector7/1, Selector6/1
  Selector6/1 -> Out1/1
  Selector23/1 -> Out7/1
  Selector2/1 -> Out3/1
  Selector18/1 -> Out9/1

== system atrias_original/control/Robot-to-NMM Interface/RC dq demux ==
  In1 : Inport
  Selector10 : Selector  InputPortWidth=13  IndexOptions=Index vector (dialog)  Indices=[7 8]  OutputSizes=1
  Selector11 : Selector  InputPortWidth=13  IndexOptions=Index vector (dialog)  Indices=[9]  OutputSizes=1
  Selector12 : Selector  InputPortWidth=13  IndexOptions=Index vector (dialog)  Indices=[1 2]  OutputSizes=1
  Selector13 : Selector  InputPortWidth=13  IndexOptions=Index vector (dialog)  Indices=[3 4]  OutputSizes=1
  Selector20 : Selector  InputPortWidth=13  IndexOptions=Index vector (dialog)  Indices=[13]  OutputSizes=1
  Selector21 : Selector  InputPortWidth=13  IndexOptions=Index vector (dialog)  Indices=[11]  OutputSizes=1
  Selector22 : Selector  InputPortWidth=13  IndexOptions=Index vector (dialog)  Indices=[12]  OutputSizes=1
  Selector8 : Selector  InputPortWidth=13  IndexOptions=Index vector (dialog)  Indices=[10]  OutputSizes=1
  Selector9 : Selector  InputPortWidth=13  IndexOptions=Index vector (dialog)  Indices=[5 6]  OutputSizes=1
  Out1 : Outport
  Out2 : Outport  Port=2
  Out3 : Outport  Port=3
  Out4 : Outport  Port=4
  Out5 : Outport  Port=5
  Out6 : Outport  Port=6
  Out7 : Outport  Port=7
  Out8 : Outport  Port=8
  Out9 : Outport  Port=9
  wires:
  Selector21/1 -> Out7/1
  Selector22/1 -> Out8/1
  Selector12/1 -> Out1/1
  Selector9/1 -> Out3/1
  In1/1 -> Selector9/1, Selector10/1, Selector11/1, Selector8/1, Selector21/1, Selector22/1, Selector20/1, Selector12/1, Selector13/1
  Selector20/1 -> Out9/1
  Selector10/1 -> Out4/1
  Selector13/1 -> Out2/1
  Selector8/1 -> Out6/1
  Selector11/1 -> Out5/1

== system atrias_original/control/Virtual Neuromuscular Control/Higher Control Layer ==
  note: Target Foot Placement
  note: Target Swing Leg Length
      | (constant)
  note: Stance to Swing Leg Decision
  note: Target Trunk Angle
      | (constant)
  note: Higher Control Layer
      | (Supra Spinal Control)
  Double Support : Subsystem
  Mux{1..4} (4 alike) : Mux  Inputs=2
  Sum{1..4} (4 alike) : Sum  Inputs=-+|
  left alpha_tgt (sagittal) : Fcn  Expr=u(1) + u(2)*u(4) + u(3)*u(5)
  right alpha_tgt (sagittal) : Fcn  Expr=u(1) + u(2)*u(4) + u(3)*u(5)
  tag scope: Lalpha_tgt=global, LonR=global, Ralpha_tgt=global, RonL=global, double_support=global, flight=global, flight_LonR=global, flight_RonL=global, leg_clr=global, theta_tgt=global
  wires:
  left alpha_tgt (sagittal)/1 -> [Lalpha_tgt]
  right alpha_tgt (sagittal)/1 -> [Ralpha_tgt]
  [LLCtrlPar] -> [leg_clr]
  Double Support/3(LonR) -> [LonR]
  [LStance] -> Double Support/1(LStance)
  [RStance] -> Double Support/2(RStance)
  Double Support/1(RonL) -> [RonL]
  Double Support/2(Flight) -> [flight]
  Sum1/1 -> Double Support/3(Lalpha_tgt)
  [Lphi23] -> Double Support/4(Lphi34)
  [Rphi23] -> Double Support/7(Rphi34)
  [Lphi12] -> Double Support/5(Lphi23)
  [Rphi12] -> Double Support/8(Rphi23)
  [Lalpha_tgt] -> Sum1/2
  [theta] -> Sum1/1, Sum2/1
  [Ralpha_tgt] -> Sum2/2
  [theta0] -> [theta_tgt]
  Mux1/1 -> left alpha_tgt (sagittal)/1
  [FPCtrlPar] -> Mux4/1, Mux1/1
  Mux2/1 -> Mux1/2
  Mux4/1 -> right alpha_tgt (sagittal)/1
  Mux3/1 -> Mux4/2
  [xRShank1] -> Sum3/1
  [xTorso] -> Sum3/2, Sum4/2
  Sum3/1 -> Mux2/1
  [xLShank1] -> Sum4/1
  Sum4/1 -> Mux3/1
  [dxTorso] -> Mux3/2, Mux2/2
  Double Support/4(DS) -> [double_support]
  Sum2/1 -> Double Support/6(Ralpha_tgt)
  Double Support/5(RonL (Flight)) -> [flight_RonL]
  Double Support/6(LonR (Flight)) -> [flight_LonR]

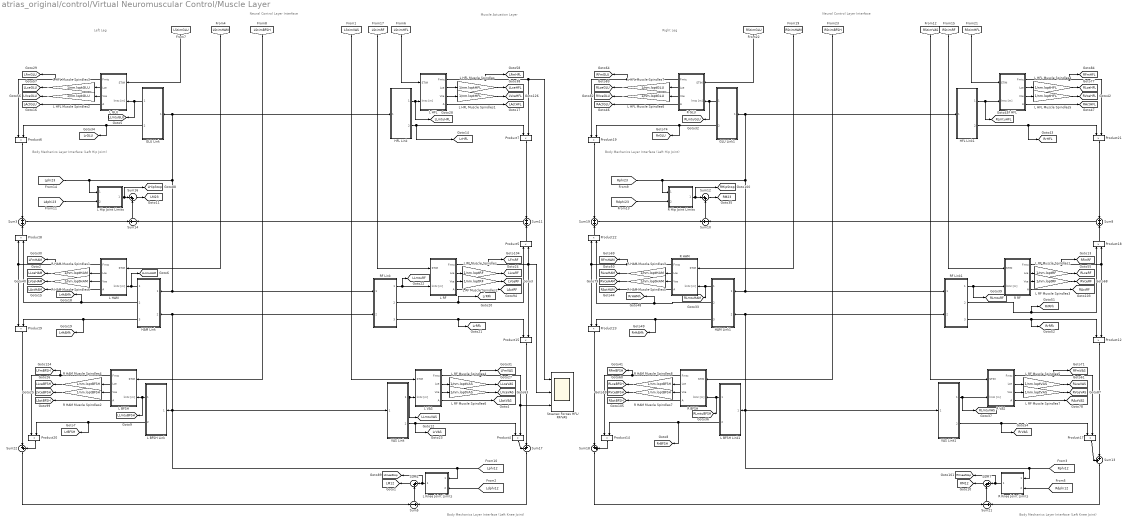
== system atrias_original/control/Virtual Neuromuscular Control/Muscle Layer ==
  note: Left Leg
  note: Neural Control Layer Interface
  note: Muscle Actuation Layer
  note: Body Mechanics Layer
      | Interface (Left Hip Joint)
  note: Body Mechanics Layer
      | Interface (Left Knee Joint)
  note: Right Leg
  note: Neural Control Layer Interface
  note: Body Mechanics Layer
      | Interface (Left Hip Joint)
  note: Body Mechanics Layer
      | Interface (Left Knee Joint)
  GLU Link : Subsystem
  GLU Link1 : Subsystem
  HAM Link : Subsystem
  HAM Link1 : Subsystem
  HFL Link : Subsystem
  HFL Link1 : Subsystem
  L BFSH : Subsystem
  L BFSH Link : Subsystem
  L BFSH Link1 : Subsystem
  L GLU : Subsystem
  L HAM : Subsystem
  L HFL : Subsystem
  L HFL Muscle Spindles{,1,4..5} (4 alike) : Gain  Gain=1/nm.loptHFL
  L HFL Muscle Spindles{2..3,6..7} (4 alike) : Gain  Gain=1/nm.loptGLU
  L Hip Joint Limits : Subsystem
  L Knee Joint Limits : Subsystem
  L RF : Subsystem
  L RF Muscle Spindles{,1..3} (4 alike) : Gain  Gain=1/nm.loptRF
  L RF Muscle Spindles{4..7} (4 alike) : Gain  Gain=1/nm.loptVAS
  L VAS : Subsystem
  Product{4..9,12,14..15,17..23} (16 alike) : Product  RndMeth=Zero
  R BFSH : Subsystem
  R GLU : Subsystem
  R HAM : Subsystem
  R HAM Muscle Spindles{1,3,5..6} (4 alike) : Gain  Gain=1/nm.loptHAM
  R HAM Muscle Spindles{2,4,7..8} (4 alike) : Gain  Gain=1/nm.loptBFSH
  R HFL : Subsystem
  R Hip Joint Limits : Subsystem
  R Knee Joint Limits : Subsystem
  R RF : Subsystem
  R VAS : Subsystem
  RF Link : Subsystem
  RF Link1 : Subsystem
  Stsanec Forces HFL/ RF/VAS : Scope  NumInputPorts=3
  Sum{1,7,12,16,18,22} (6 alike) : Sum  Inputs=|++
  Sum10 : Sum  Inputs=+-
  Sum{3,8,11,19} (4 alike) : Sum
  Sum13 : Sum  Inputs=++|
  Sum14 : Sum  Inputs=+-
  Sum17 : Sum  Inputs=++|
  Sum21 : Sum  Inputs=-+
  Sum5 : Sum  Inputs=-+
  VAS Link : Subsystem
  VAS Link1 : Subsystem
  tag scope: LActBFSH=global, LActGLU=global, LActHAM=global, LActHFL=global, LActRF=global, LActVAS=global, LFmBFSH=global, LFmGLU=global, LFmHAM=global, LFmHFL=global, LFmRF=global, LFmVAS=global, LHipStop=global, LKneeStop=global, LLceBFSH=global, LLceGLU=global, LLceHAM=global, LLceHFL=global, LLceRF=global, LLceVAS=global, LLmtuBFSH=global, LLmtuGLU=global, LLmtuHAM=global, LLmtuHFL=global, LLmtuRF=global, LLmtuVAS=global, LM12=global, LM23=global, LVceBFSH=global, LVceGLU=global, LVceHAM=global, LVceHFL=global, LVceRF=global, LVceVAS=global, LrBFSH=global, LrGLU=global, LrHAMh=global, LrHAMk=global, LrHFL=global, LrRFh=global, LrRFk=global, LrVAS=global, RActBFSH=global, RActGLU=global, RActHAM=global, RActHFL=global, RActRF=global, RActVAS=global, RFmBFSH=global, RFmGLU=global, RFmHAM=global, RFmHFL=global, RFmRF=global, RFmVAS=global, RHipStop=global, RKneeStop=global, RLceBFSH=global, RLceGLU=global, RLceHAM=global, RLceHFL=global, RLceRF=global, RLceVAS=global, RLmtuBFSH=global, RLmtuGLU=global, RLmtuHAM=global, RLmtuHFL=global, RLmtuRF=global, RLmtuVAS=global, RM12=global, RM23=global, RVceBFSH=global, RVceGLU=global, RVceHAM=global, RVceHFL=global, RVceRF=global, RVceVAS=global, RrBFSH=global, RrGLU=global, RrHAMh=global, RrHAMk=global, RrHFL=global, RrRFh=global, RrRFk=global, RrVAS=global
  wires:
  [Lphi12] -> L Knee Joint Limits/1(phi [rad]), VAS Link/1(phi23 [rad]), RF Link/2(phi23 [rad]), HAM Link/2(phi23 [rad]), L BFSH Link/1(phi23 [rad])
  [LStimHAM] -> L HAM/1(STIM)
  L HAM/1(Fmtc) -> Product9/1, Product8/1, [LFmHAM]
  L HAM/2(Lce) -> R HAM Muscle Spindles1/1
  L HFL/1(Fmtc) -> Product7/2, Stsanec Forces HFL/ RF/VAS/1, [LFmHFL]
  L HFL/2(Lce) -> L HFL Muscle Spindles/1
  [LStimHFL] -> L HFL/1(STIM)
  L GLU/1(Fmtc) -> Product6/1, [LFmGLU]
  [LStimGLU] -> L GLU/1(STIM)
  Sum16/1 -> [LM23]
  [Ldphi12] -> L Knee Joint Limits/2(dphi [rad/s])
  VAS Link/1(lmtu [m]) -> L VAS/2(lmtc [m]), [LLmtuVAS]
  HAM Link/1(lmtu [m]) -> L HAM/2(lmtc [m]), [LLmtuHAM]
  HAM Link/2(lever34 [m]) -> Product8/2, [LrHAMh]
  HAM Link/3(lever23 [m]) -> Product9/2, [LrHAMk]
  Sum3/1 -> Sum14/1
  [Lphi23] -> L Hip Joint Limits/1(phi [rad]), HFL Link/1(phi34 [rad]), GLU Link/1(phi34 [rad]), HAM Link/1(phi34 [rad]), RF Link/1(phi34 [rad])
  L VAS/4(A) -> [LActVAS]
  L VAS/1(Fmtc) -> Stsanec Forces HFL/ RF/VAS/3, Product4/2, [LFmVAS]
  Sum1/1 -> [LM12]
  L Knee Joint Limits/1(M_stop [Nm]) -> Sum1/1, [LKneeStop]
  Sum5/1 -> Sum1/2
  VAS Link/2(lever [m]) -> [LrVAS], Product4/1
  Sum22/1 -> Sum5/1
  L HAM/4(A) -> [LActHAM]
  Product8/1 -> Sum3/2
  Product6/1 -> Sum3/1
  GLU Link/1(lmtu [m]) -> [LLmtuGLU], L GLU/2(lmtc [m])
  GLU Link/2(lever [m]) -> Product6/2, [LrGLU]
  L GLU/4(A) -> [LActGLU]
  [Ldphi23] -> L Hip Joint Limits/2(dphi [rad/s])
  L Hip Joint Limits/1(M_stop [Nm]) -> [LHipStop], Sum16/1
  Sum14/1 -> Sum16/2
  HFL Link/1(lmtu [m]) -> [LLmtuHFL], L HFL/2(lmtc [m])
  L HFL/4(A) -> [LActHFL]
  HFL Link/2(lever [m]) -> Product7/1, [LrHFL]
  [LStimVAS] -> L VAS/1(STIM)
  L GLU/2(Lce) -> L HFL Muscle Spindles3/1
  L GLU/3(Vce) -> L HFL Muscle Spindles2/1
  L HAM/3(Vce) -> R HAM Muscle Spindles6/1
  L VAS/3(Vce) -> L RF Muscle Spindles6/1
  L VAS/2(Lce) -> L RF Muscle Spindles4/1
  L HFL/3(Vce) -> L HFL Muscle Spindles1/1
  L RF/4(A) -> [LActRF]
  L RF/3(Vce) -> L RF Muscle Spindles2/1
  L RF/2(Lce) -> L RF Muscle Spindles/1
  RF Link/1(lmtu [m]) -> L RF/2(lmtc [m]), [LLmtuRF]
  RF Link/2(lever34 [m]) -> Product5/1, [LrRFh]
  RF Link/3(lever23 [m]) -> Product15/1, [LrRFk]
  [LStimRF] -> L RF/1(STIM)
  Product7/1 -> Sum11/1
  Product5/1 -> Sum11/2
  Product15/1 -> Sum17/2
  Sum17/1 -> Sum5/2
  Product4/1 -> Sum17/1
  [LStimBFSH] -> L BFSH/1(STIM)
  L BFSH Link/1(lmtu [m]) -> [LLmtuBFSH], L BFSH/2(lmtc [m])
  L BFSH Link/2(lever [m]) -> [LrBFSH], Product20/2
  L BFSH/4(A) -> [LActBFSH]
  L BFSH/2(Lce) -> R HAM Muscle Spindles4/1
  L BFSH/3(Vce) -> R HAM Muscle Spindles2/1
  Product20/1 -> Sum22/2
  Product9/1 -> Sum22/1
  L HFL Muscle Spindles1/1 -> [LVceHFL]
  L HFL Muscle Spindles2/1 -> [LVceGLU]
  L HFL Muscle Spindles3/1 -> [LLceGLU]
  L RF Muscle Spindles6/1 -> [LVceVAS]
  L RF/1(Fmtc) -> Stsanec Forces HFL/ RF/VAS/2, Product5/2, Product15/2, [LFmRF]
  L BFSH/1(Fmtc) -> Product20/1, [LFmBFSH]
  L HFL Muscle Spindles/1 -> [LLceHFL]
  R HAM Muscle Spindles1/1 -> [LLceHAM]
  R HAM Muscle Spindles6/1 -> [LVceHAM]
  L RF Muscle Spindles/1 -> [LLceRF]
  L RF Muscle Spindles2/1 -> [LVceRF]
  R HAM Muscle Spindles4/1 -> [LLceBFSH]
  R HAM Muscle Spindles2/1 -> [LVceBFSH]
  L RF Muscle Spindles4/1 -> [LLceVAS]
  [Rphi12] -> R Knee Joint Limits/1(phi [rad]), VAS Link1/1(phi23 [rad]), L BFSH Link1/1(phi23 [rad]), RF Link1/2(phi23 [rad]), HAM Link1/2(phi23 [rad])
  [RStimHAM] -> R HAM/1(STIM)
  R HAM/1(Fmtc) -> Product23/1, Product22/1, [RFmHAM]
  R HAM/2(Lce) -> R HAM Muscle Spindles3/1
  R HFL/1(Fmtc) -> [RFmHFL], Product21/2
  R HFL/2(Lce) -> L HFL Muscle Spindles4/1
  [RStimHFL] -> R HFL/1(STIM)
  R GLU/1(Fmtc) -> Product19/1, [RFmGLU]
  [RStimGLU] -> R GLU/1(STIM)
  Sum12/1 -> [RM23]
  [Rdphi12] -> R Knee Joint Limits/2(dphi [rad/s])
  VAS Link1/1(lmtu [m]) -> R VAS/2(lmtc [m]), [RLmtuVAS]
  HAM Link1/1(lmtu [m]) -> R HAM/2(lmtc [m]), [RLmtuHAM]
  HAM Link1/2(lever34 [m]) -> Product22/2, [RrHAMh]
  HAM Link1/3(lever23 [m]) -> Product23/2, [RrHAMk]
  Sum19/1 -> Sum10/1
  [Rphi23] -> R Hip Joint Limits/1(phi [rad]), HFL Link1/1(phi34 [rad]), GLU Link1/1(phi34 [rad]), RF Link1/1(phi34 [rad]), HAM Link1/1(phi34 [rad])
  R VAS/4(A) -> [RActVAS]
  R VAS/1(Fmtc) -> Product17/2, [RFmVAS]
  Sum7/1 -> [RM12]
  R Knee Joint Limits/1(M_stop [Nm]) -> Sum7/1, [RKneeStop]
  Sum21/1 -> Sum7/2
  VAS Link1/2(lever [m]) -> [RrVAS], Product17/1
  Sum18/1 -> Sum21/1
  R HAM/4(A) -> [RActHAM]
  Product22/1 -> Sum19/2
  Product19/1 -> Sum19/1
  GLU Link1/1(lmtu [m]) -> R GLU/2(lmtc [m]), [RLmtuGLU]
  GLU Link1/2(lever [m]) -> Product19/2, [RrGLU]
  R GLU/4(A) -> [RActGLU]
  [Rdphi23] -> R Hip Joint Limits/2(dphi [rad/s])
  R Hip Joint Limits/1(M_stop [Nm]) -> [RHipStop], Sum12/1
  Sum10/1 -> Sum12/2
  HFL Link1/1(lmtu [m]) -> [RLmtuHFL], R HFL/2(lmtc [m])
  R HFL/4(A) -> [RActHFL]
  HFL Link1/2(lever [m]) -> Product21/1, [RrHFL]
  [RStimVAS] -> R VAS/1(STIM)
  R GLU/2(Lce) -> L HFL Muscle Spindles7/1
  R GLU/3(Vce) -> L HFL Muscle Spindles6/1
  R HAM/3(Vce) -> R HAM Muscle Spindles5/1
  R VAS/3(Vce) -> L RF Muscle Spindles7/1
  R VAS/2(Lce) -> L RF Muscle Spindles5/1
  R HFL/3(Vce) -> L HFL Muscle Spindles5/1
  R RF/4(A) -> [RActRF]
  R RF/3(Vce) -> L RF Muscle Spindles3/1
  R RF/2(Lce) -> L RF Muscle Spindles1/1
  RF Link1/1(lmtu [m]) -> R RF/2(lmtc [m]), [RLmtuRF]
  RF Link1/2(lever34 [m]) -> Product18/1, [RrRFh]
  RF Link1/3(lever23 [m]) -> [RrRFk], Product12/1
  [RStimRF] -> R RF/1(STIM)
  Sum8/1 -> Sum10/2
  Product21/1 -> Sum8/1
  Product18/1 -> Sum8/2
  Product12/1 -> Sum13/2
  Sum13/1 -> Sum21/2
  Product17/1 -> Sum13/1
  [RStimBFSH] -> R BFSH/1(STIM)
  L BFSH Link1/1(lmtu [m]) -> R BFSH/2(lmtc [m]), [RLmtuBFSH]
  L BFSH Link1/2(lever [m]) -> [RrBFSH], Product14/2
  R BFSH/4(A) -> [RActBFSH]
  R BFSH/2(Lce) -> R HAM Muscle Spindles8/1
  R BFSH/3(Vce) -> R HAM Muscle Spindles7/1
  Product14/1 -> Sum18/2
  Product23/1 -> Sum18/1
  L HFL Muscle Spindles5/1 -> [RVceHFL]
  L HFL Muscle Spindles6/1 -> [RVceGLU]
  L HFL Muscle Spindles7/1 -> [RLceGLU]
  L RF Muscle Spindles7/1 -> [RVceVAS]
  R RF/1(Fmtc) -> Product18/2, Product12/2, [RFmRF]
  R BFSH/1(Fmtc) -> Product14/1, [RFmBFSH]
  L HFL Muscle Spindles4/1 -> [RLceHFL]
  R HAM Muscle Spindles3/1 -> [RLceHAM]
  R HAM Muscle Spindles5/1 -> [RVceHAM]
  L RF Muscle Spindles1/1 -> [RLceRF]
  L RF Muscle Spindles3/1 -> [RVceRF]
  R HAM Muscle Spindles8/1 -> [RLceBFSH]
  R HAM Muscle Spindles7/1 -> [RVceBFSH]
  L RF Muscle Spindles5/1 -> [RLceVAS]
  Sum11/1 -> Sum14/2
